simulink model "Obstacle_Avoiding_Robot_v2018a"  (R2018a)
settings: Solver=FixedStepAuto  StartTime=0.0  StopTime=inf  RelTol=1e-3  EnableMultiTasking=on
libraries: arduinolib x4, LCDlib x1, arduinosensorlib x1
settings Model: SimulationMode=external  ExtModeTrigDuration=2  Creator=Shyam lal  LastModifiedBy=Shyam lal
settings DataIOCC: ReturnWorkspaceOutputs=on
settings OptimizationCC: EnhancedBackFolding=on  PassReuseOutputArgsAs=Individual arguments  MaxStackSize=64  OptimizeBlockOrder=speed  DifferentSizesBufferReuse=on  OptimizationCustomize=off
settings DebuggingCC: ParameterTunabilityLossMsg=error
settings HardwareCC: ProdBitPerInt=16  ProdBitPerPointer=16  ProdBitPerSizeT=16  ProdBitPerPtrDiffT=16  ProdLargestAtomicFloat=None  ProdWordSize=8  ProdHWDeviceType=Atmel->AVR
settings SFSimCC: SimUseLocalCustomCode=on  MATLABDynamicMemAlloc=off
settings RTWCC: SystemTargetFile=ert.tlc  HardwareBoard=Arduino Uno  TLCOptions=-aInlineSetEventsForThisBaseRateFcn=TLC_FALSE -aSuppressMultiTaskScheduler=TLC_FALSE -aRateBasedStepFcn=1  TemplateMakefile=ert_default_tmf  GenerateReport=on  RTWUseLocalCustomCode=on  Toolchain=Arduino AVR  BuildConfiguration=Faster Runs  IncludeHyperlinkInReport=on  LaunchReport=on  GenerateTraceInfo=on  GenerateTraceReport=on  GenerateTraceReportSl=on  GenerateTraceReportSf=on  GenerateTraceReportEml=on
settings CodeAppCC: ForceParamTrailComments=on  IgnoreCustomStorageClasses=off  OperatorAnnotations=on  SimulinkDataObjDesc=on  SFDataObjDesc=on  InsertBlockDesc=on
settings ERTTargetCC: SupportContinuousTime=on  SupportVariableSizeSignals=on  ExtModeStaticAllocSize=250

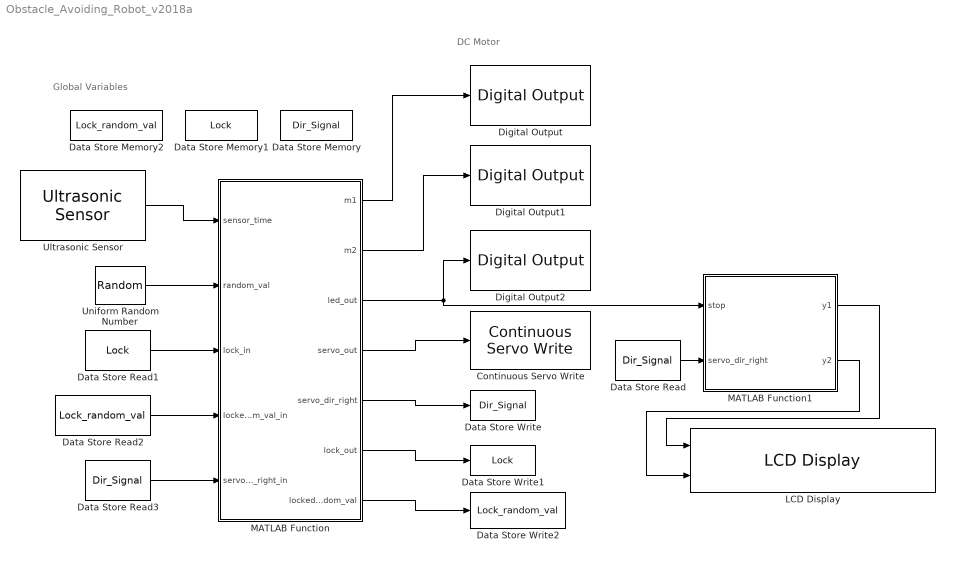
== system Obstacle_Avoiding_Robot_v2018a ==
  note: DC Motor
  note: Global Variables
  Continuous Servo Write : arduinolib/Continuous Servo Write  pinNumber=12  ServoIndex=0  blockPlatform=ARDUINO
      settings: SourceProductName=Simulink Support Package for Arduino Hardware  SourceProductBaseCode=ARDUINO
  Data Store Memory : DataStoreMemory  DataStoreName=Dir_Signal  ReadBeforeWriteMsg=warning  WriteAfterWriteMsg=warning  WriteAfterReadMsg=warning  ShowAdditionalParam=off
  Data Store Memory1 : DataStoreMemory  DataStoreName=Lock  ReadBeforeWriteMsg=warning  WriteAfterWriteMsg=warning  WriteAfterReadMsg=warning  ShowAdditionalParam=off
  Data Store Memory2 : DataStoreMemory  DataStoreName=Lock_random_val  ReadBeforeWriteMsg=warning  WriteAfterWriteMsg=warning  WriteAfterReadMsg=warning  ShowAdditionalParam=off
  Data Store Read : DataStoreRead  DataStoreName=Dir_Signal
  Data Store Read1 : DataStoreRead  DataStoreName=Lock
  Data Store Read2 : DataStoreRead  DataStoreName=Lock_random_val
  Data Store Read3 : DataStoreRead  DataStoreName=Dir_Signal
  Data Store Write : DataStoreWrite  DataStoreName=Dir_Signal
  Data Store Write1 : DataStoreWrite  DataStoreName=Lock
  Data Store Write2 : DataStoreWrite  DataStoreName=Lock_random_val
  Digital Output : arduinolib/Digital Output  pinNumber=4  blockPlatform=arduino
  Digital Output1 : arduinolib/Digital Output  pinNumber=5  blockPlatform=arduino
  Digital Output2 : arduinolib/Digital Output  pinNumber=13  blockPlatform=arduino
  LCD Display : LCDlib/LCD Display  pins=[6,7,8,9,10,11]
      settings: SourceProductName=LCD Library
  MATLAB Function : MATLAB Function  TreatAsAtomicUnit=on
  MATLAB Function1 : MATLAB Function  TreatAsAtomicUnit=on
  Ultrasonic Sensor : arduinosensorlib/Ultrasonic Sensor  NumSignalPins=2  TrigPin=2  EchoPin=3  SignalPin=3  SampleTime_=0.1  blockPlatform=ARDUINO
      settings: SourceProductName=Simulink Support Package for Arduino Hardware  SourceProductBaseCode=ARDUINO
  Uniform Random Number : UniformRandomNumber  SampleTime=0.1
  wires:
  Ultrasonic Sensor/1 -> MATLAB Function/1(sensor_time)
  MATLAB Function1/1(y1) -> LCD Display/1
  MATLAB Function1/2(y2) -> LCD Display/2
  MATLAB Function/4(servo_out) -> Continuous Servo Write/1
  MATLAB Function/3(led_out) -> Digital Output2/1, MATLAB Function1/1(stop)
  MATLAB Function/5(servo_dir_right) -> Data Store Write/1
  Data Store Read/1 -> MATLAB Function1/2(servo_dir_right)
  Uniform Random Number/1 -> MATLAB Function/2(random_val)
  Data Store Read1/1 -> MATLAB Function/3(lock_in)
  Data Store Read2/1 -> MATLAB Function/4(locked_random_val_in)
  MATLAB Function/7(locked_random_val) -> Data Store Write2/1
  MATLAB Function/6(lock_out) -> Data Store Write1/1
  Data Store Read3/1 -> MATLAB Function/5(servo_dir_right_in)
  MATLAB Function/2(m2) -> Digital Output1/1
  MATLAB Function/1(m1) -> Digital Output/1

== matlab function Obstacle_Avoiding_Robot_v2018a/MATLAB Function1 ==
  data: stop input; y1 output; y2 output; servo_dir_right input
function [y1,y2] = fcn(stop, servo_dir_right)
if ~stop
    y1=[[68], [67], [32], [77], [111], [116], [111], [114], [32], [82], [80], [77], [58], [32]];
    y2=[[51], [48], [48], [32], [32], [32], [32], [32], [32], [32], [32], [32], [32], [32]];
else
    y1=[[65], [76], [69], [82], [84], [33], [33], [32], [32], [32], [32], [32], [32], [32]];
    if servo_dir_right
        y2=[[84], [117], [114], [110], [105], [110], [103], [32], [76], [101], [102], [116], [46], [32]];
    else
        y2=[[84], [117], [114], [110], [105], [110], [103], [32], [82], [105], [103], [104], [116], [46]];
    end
end
end

== matlab function Obstacle_Avoiding_Robot_v2018a/MATLAB Function ==
  data: sensor_time input; m1 output; m2 output; led_out output; servo_out output; random_val input; servo_dir_right output; lock_out output; locked_random_val output; lock_in input; locked_random_val_in input; servo_dir_right_in input
function [m1,m2,led_out,servo_out,servo_dir_right, lock_out,locked_random_val] = fcn(sensor_time, random_val, lock_in, locked_random_val_in, servo_dir_right_in)
distance=(sensor_time*343)/2;
if distance < 20
    m1=0;
    m2=0;
    led_out=1;
    if lock_in==0
        locked_random_val=random_val;
        servo_dir_right=servo_dir_right_in;
        servo_out=[0];
    else
        locked_random_val=locked_random_val_in;
        if locked_random_val_in>0
            servo_out=[90];
            servo_dir_right=1;
        else
            servo_out=[-90];
            servo_dir_right=0;
        end
    end
    lock_out=1;
else
    m1=1;
    m2=0;
    led_out=0;
    servo_out=[0];
    locked_random_val=locked_random_val_in;
    servo_dir_right=servo_dir_right_in;
    lock_out=0;
end
% if locked_random_val_in>0
%     servo_dir_right=1;
% else
%     servo_dir_right=0;
% end
end
